simulink model "firstordersys"  (R2015a)
settings: Solver=ode45  StartTime=0.0  StopTime=10.0  RelTol=1e-3
libraries: cstblocks x3, simulink x1
settings Model: Creator=LENOVO  LastModifiedBy=LENOVO

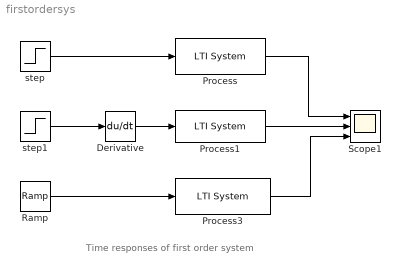
== system firstordersys ==
  note: Time responses of first order system
  Derivative : Derivative
  Process : cstblocks/LTI System  sys=tf(5,[0.5 1])  IC=[]
  Process1 : cstblocks/LTI System  sys=tf(5,[0.5 1])  IC=[]
  Process3 : cstblocks/LTI System  sys=tf(5,[0.5 1])  IC=[]
  Ramp : simulink/Sources/Ramp  slope=1  start=0  X0=0
  Scope1 : Scope  NumInputPorts=3
      settings: TickLabels=on  TimeRange=10  YMin=0~0~0  YMax=5~0.3~50
  step : Step  Time=0  SampleTime=0
  step1 : Step  Time=0.01  SampleTime=0
  wires:
  step/1 -> Process/1
  step1/1 -> Derivative/1
  Derivative/1 -> Process1/1
  Process1/1 -> Scope1/2
  Process/1 -> Scope1/1
  Process3/1 -> Scope1/3
  Ramp/1 -> Process3/1
